simulink model "OL"  (R2025b)
settings: Solver=VariableStepAuto  StartTime=0.0  StopTime=10.0  RelTol=1e-3
values from neighbouring files (symbols this model uses):
  plant = ss(a,b,c,d)    [data_avion_lat.m]
settings Model: Creator=flo  LastModifiedBy=flo

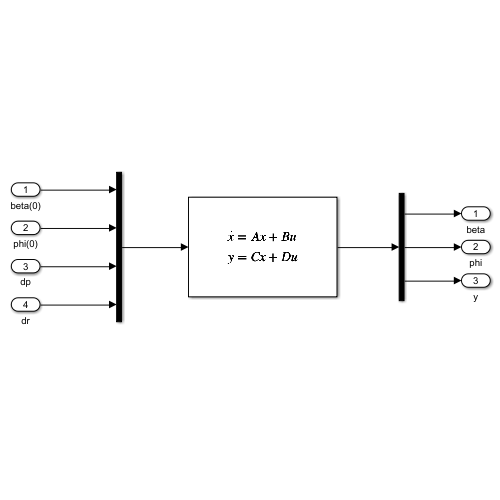
[thumbnail: Simulink's stored preview of the top-level diagram]
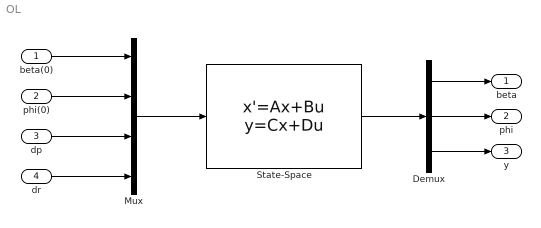
== system OL ==
  beta(0) : Inport
  phi(0) : Inport  Port=2
  dp : Inport  Port=3
  dr : Inport  Port=4
  Demux : Demux  Outputs=[1;1;4]
  Mux : Mux
  State-Space : StateSpace  A=plant.a  B=[[1 0; 0 0; 0 0; 0 1] plant.b]  C=[[1 0 0 0; 0 0 0 1]; plant.c]  D=[zeros(2,4); zeros(4,2) plant.d]  InitialCondition=0
  beta : Outport
  phi : Outport  Port=2
  y : Outport  Port=3
  wires:
  Mux/1 -> State-Space/1
  beta(0)/1 -> Mux/1
  phi(0)/1 -> Mux/2
  dp/1 -> Mux/3
  dr/1 -> Mux/4
  State-Space/1 -> Demux/1
  Demux/2 -> phi/1
  Demux/1 -> beta/1
  Demux/3 -> y/1
